simulink model "pnseq"  (R2022a)
settings: Solver=VariableStepAuto  StartTime=0.0  StopTime=10.0  RelTol=1e-3
settings Model: Creator=S&S LAB  LastModifiedBy=Sanil Sattarkar
settings SolverCC: AlgebraicLoopSolver=TrustRegion
settings DebuggingCC: UnconnectedInputMsg=warning  UnconnectedOutputMsg=warning  UnconnectedLineMsg=warning  SFMachineParentedDataDiag=warning
settings SFSimCC: CustomCodeUndefinedFunction=UseInterfaceOnly

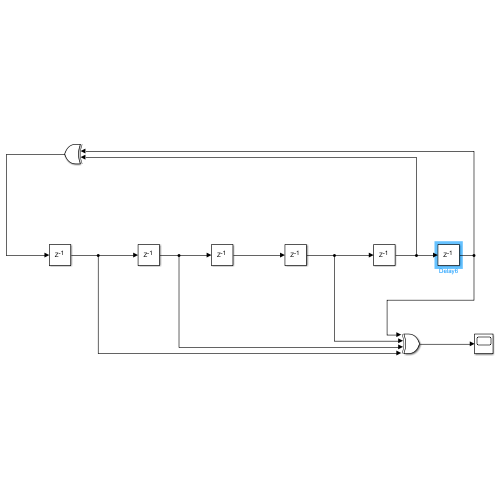
[thumbnail: Simulink's stored preview of the top-level diagram]
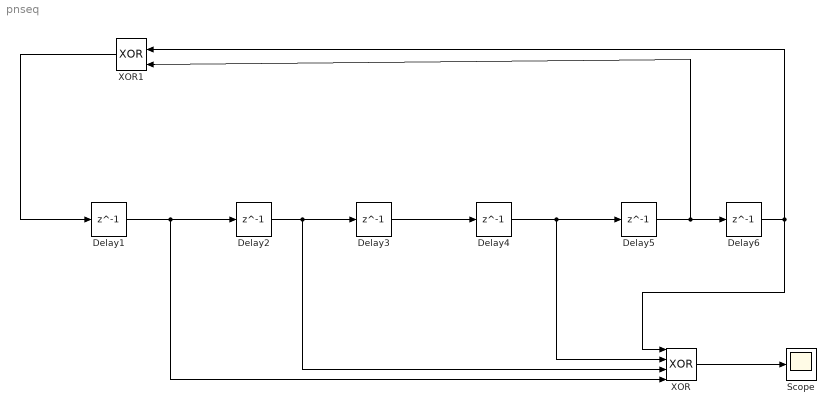
== system pnseq ==
  Delay1 : Delay  DelayLength=1  InitialCondition=0001
  Delay2 : Delay  DelayLength=1  InitialCondition=0010
  Delay3 : Delay  DelayLength=1  InitialCondition=0100
  Delay4 : Delay  DelayLength=1  InitialCondition=1000
  Delay5 : Delay  DelayLength=1  InitialCondition=1001
  Delay6 : Delay  DelayLength=1  InitialCondition=1010
  Scope : Scope
  XOR : Logic  Operator=XOR  Inputs=4  IconShape=distinctive  AllPortsSameDT=off  OutDataTypeStr=boolean
  XOR1 : Logic  Operator=XOR  IconShape=distinctive  AllPortsSameDT=off  OutDataTypeStr=boolean
  wires:
  XOR1/1 -> Delay1/1
  Delay1/1 -> XOR/4, Delay2/1
  Delay2/1 -> XOR/3, Delay3/1
  Delay3/1 -> Delay4/1
  Delay4/1 -> XOR/2, Delay5/1
  Delay5/1 -> XOR1/2, Delay6/1
  Delay6/1 -> XOR/1, XOR1/1
  XOR/1 -> Scope/1
